simulink model "read_write_sl"  (R2020b)
settings: Solver=VariableStepAuto  StartTime=0.0  StopTime=10.0  RelTol=1e-3
settings Model: Creator=johnc  LastModifiedBy=johnc
settings SFSimCC: SimCustomHeaderCode="#include \"dynamixel_sdk.h\""
settings SFSimCC: SimUserIncludeDirs=|
  | C:\Users\johnc\OneDrive\Documentos\DYNAMIXEL\DynamixelSDK-3.7.31\c\include\dynamixel_sdk\
  | C:\Users\johnc\OneDrive\Documentos\DYNAMIXEL\DynamixelSDK-3.7.31\c\build\win32\output\
  | C:\Users\johnc\OneDrive\Documentos\DYNAMIXEL\DynamixelSDK-3.7.31\c\build\win64\output\
  | C:\Users\johnc\OneDrive\Documentos\DYNAMIXEL\DynamixelSDK-3.7.31\c\src\dynamixel_sdk\
settings SFSimCC: SimUserLibraries=|
  | dxl_x86_c.dll
  | dxl_x64_c.dll
settings SFSimCC: SimUserDefines=|
  | _WIN32
  | _WIN64
  | _cplusplus
  | size_t=unsigned __int64
  | size_t=unsigned in

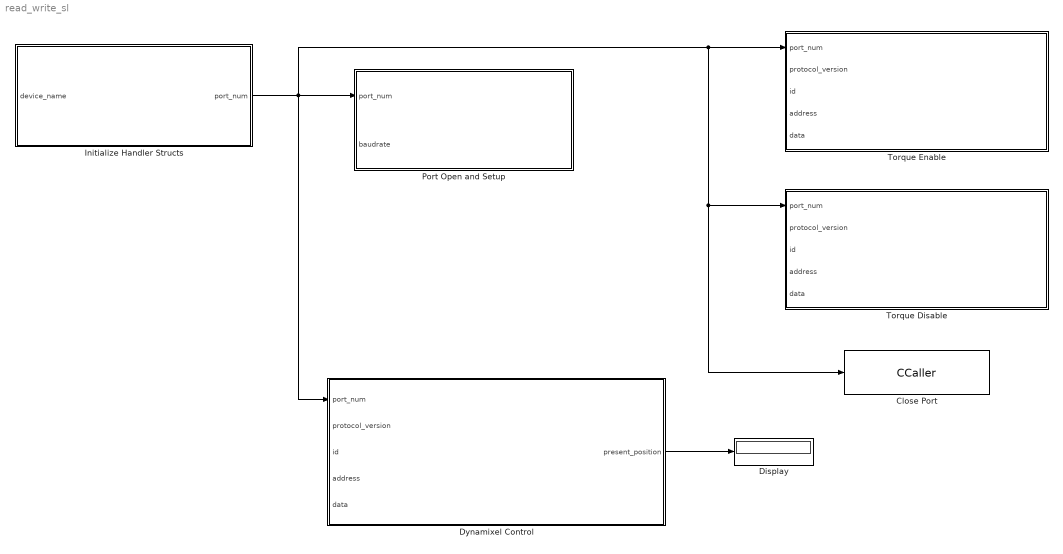
== system read_write_sl ==
  Close Port : CCaller  FunctionName=closePort  PortSpecificationStruct="%)30     .    * (   8    (     @         %    \"     $    !     0         %  0 \"0    $    _    07)G3F%M90  4&]R=$YA;64 4V-O<&4     26YD97@     5'EP90      4VEZ90      27-';&]B86P   X    X    !@    @    $          4    (     0    @    !         !     (    <&]R=%]N=6T.    .     8    (    !          %    \"     $    (     0         0    \"    '!O<G1?;G5M#@   #@    &    \"     0         !0    @    !    !0    $         $     4   !);G!U=     X    X    !@    @    &          4    (     0    $    !          D    (               .    .     8    (    !          %    \"     $    %     0         0    !0   &EN=#,R    #@   #     &    \"     0         !0    @    !     0    $         $  ! #$    .    ,     8    (    \"0(        %    \"     $    !     0         \"  $"
  Display : Display
  Dynamixel Control : Subsystem
  Initialize Handler Structs : Subsystem
  Port Open and Setup : Subsystem
  Torque Disable : Subsystem
  Torque Enable : Subsystem
  wires:
  Initialize Handler Structs/1(port_num) -> Port Open and Setup/1(port_num), Close Port/1, Torque Disable/1(port_num), Torque Enable/1(port_num), Dynamixel Control/1(port_num)
  Dynamixel Control/1(present_position) -> Display/1

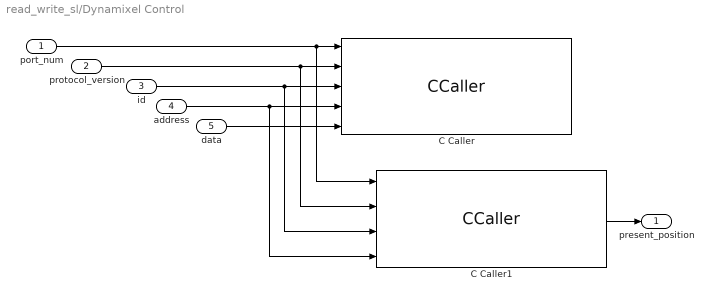
== system read_write_sl/Dynamixel Control ==
  port_num : Inport
  protocol_version : Inport  Port=2
  id : Inport  Port=3
  address : Inport  Port=4
  data : Inport  Port=5
  C Caller : CCaller  FunctionName=write1ByteTxRx  PortSpecificationStruct="%)30     .    V @   8    (     @         %    \"     4    !     0         %  0 \"0    $    _    07)G3F%M90  4&]R=$YA;64 4V-O<&4     26YD97@     5'EP90      4VEZ90      27-';&]B86P   X    X    !@    @    $          4    (     0    @    !         !     (    <&]R=%]N=6T.    .     8    (    !          %    \"     $    (     0         0    \"    '!O<G1?;G5M#@   #@    &    \"     0         !0    @    !  ...(+2668 chars)"
  C Caller1 : CCaller  FunctionName=read2ByteTxRx  PortSpecificationStruct="%)30     .    V @   8    (     @         %    \"     4    !     0         %  0 \"0    $    _    07)G3F%M90  4&]R=$YA;64 4V-O<&4     26YD97@     5'EP90      4VEZ90      27-';&]B86P   X    P    !@    @    $          4    (     0    ,    !         !   P!O=70 #@   #     &    \"     0         !0    @    !     P    $         $  # &]U=  .    .     8    (    !          %    \"     $    &     0         0   ...(+2666 chars)"
  present_position : Outport
  wires:
  port_num/1 -> C Caller1/1, C Caller/1
  address/1 -> C Caller1/4, C Caller/4
  protocol_version/1 -> C Caller1/2, C Caller/2
  id/1 -> C Caller1/3, C Caller/3
  C Caller1/1 -> present_position/1
  data/1 -> C Caller/5

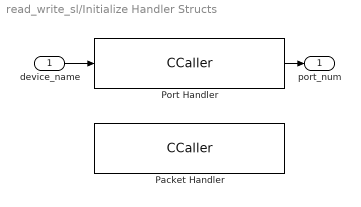
== system read_write_sl/Initialize Handler Structs ==
  device_name : Inport
  Packet Handler : CCaller  FunctionName=packetHandler
  Port Handler : CCaller  FunctionName=portHandler  PortSpecificationStruct="%)30     .    T ,   8    (     @         %    \"     (    !     0         %  0 \"0    $    _    07)G3F%M90  4&]R=$YA;64 4V-O<&4     26YD97@     5'EP90      4VEZ90      27-';&]B86P   X    P    !@    @    $          4    (     0    ,    !         !   P!O=70 #@   #     &    \"     0         !0    @    !     P    $         $  # &]U=  .    .     8    (    !          %    \"     $    &     0         0    !@   $]U='!U=   #@   #@    &    \"     8         !0    @    !     0    $         \"0    @               X    X    !@    @    $          4    (     0    4    !         !     %    :6YT,S(    .    ,     8    (    !          %    \"     $    !     0         0  $ ,0    X    P    !@    @    ) @        4    (     0    $    !          (  0      #@   $     &    \"     0         !0    @    !    \"0    $         $     D   !P;W)T7VYA;64         #@   $     &    \"     0         !0    @    !    \"0    $         $     D   !P;W)T7VYA;64         #@   #@    &    \"     0         !0    @    !    !0    $         $     4   !);G!U=     X    X    !@    @    &          4    (     0    $    !          D    (               .    ,     8    (    !          %    \"     $    $     0         0  0 :6YT. X    P    !@    @    $          4    (     0    (    !         !   @ M,0  #@   #     &    \"     D\"        !0    @    !     0    $          @ !"
  port_num : Outport
  wires:
  device_name/1 -> Port Handler/1
  Port Handler/1 -> port_num/1

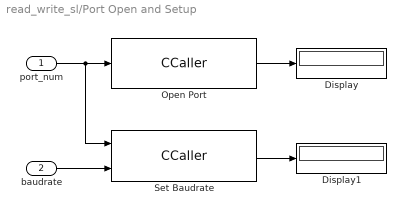
== system read_write_sl/Port Open and Setup ==
  port_num : Inport
  baudrate : Inport  Port=2
  Display : Display
  Display1 : Display
  Open Port : CCaller  FunctionName=openPort  PortSpecificationStruct="%)30     .    R ,   8    (     @         %    \"     (    !     0         %  0 \"0    $    _    07)G3F%M90  4&]R=$YA;64 4V-O<&4     26YD97@     5'EP90      4VEZ90      27-';&]B86P   X    P    !@    @    $          4    (     0    ,    !         !   P!O=70 #@   #     &    \"     0         !0    @    !     P    $         $  # &]U=  .    .     8    (    !          %    \"     $    &     0         0    !@   $]U='!U=   #@   #@    &    \"     8         !0    @    !     0    $         \"0    @               X    X    !@    @    $          4    (     0    4    !         !     %    =6EN=#@    .    ,     8    (    !          %    \"     $    !     0         0  $ ,0    X    P    !@    @    ) @        4    (     0    $    !          (  0      #@   #@    &    \"     0         !0    @    !    \"     $         $     @   !P;W)T7VYU;0X    X    !@    @    $          4    (     0    @    !         !     (    <&]R=%]N=6T.    .     8    (    !          %    \"     $    %     0         0    !0   $EN<'5T    #@   #@    &    \"     8         !0    @    !     0    $         \"0    @               X    X    !@    @    $          4    (     0    4    !         !     %    :6YT,S(    .    ,     8    (    !          %    \"     $    !     0         0  $ ,0    X    P    !@    @    ) @        4    (     0    $    !          (  0"
  Set Baudrate : CCaller  FunctionName=setBaudRate  PortSpecificationStruct="%)30     .    > 4   8    (     @         %    \"     ,    !     0         %  0 \"0    $    _    07)G3F%M90  4&]R=$YA;64 4V-O<&4     26YD97@     5'EP90      4VEZ90      27-';&]B86P   X    P    !@    @    $          4    (     0    ,    !         !   P!O=70 #@   #     &    \"     0         !0    @    !     P    $         $  # &]U=  .    .     8    (    !          %    \"     $    &     0         0    !@   $]U='!U=   #@   #@    &    \"     8         !0    @    !     0    $         \"0    @               X    X    !@    @    $          4    (     0    4    !         !     %    =6EN=#@    .    ,     8    (    !          %    \"     $    !     0         0  $ ,0    X    P    !@    @    ) @        4    (     0    $    !          (  0      #@   #@    &    \"     0         !0    @    !    \"     $         $     @   !P;W)T7VYU;0X    X    !@    @    $          4    (     0    @    !         !     (    <&]R=%]N=6T.    .     8    (    !          %    \"     $    %     0         0    !0   $EN<'5T    #@   #@    &    \"     8         !0    @    !     0    $         \"0    @               X    X    !@    @    $          4    (     0    4    !         !     %    :6YT,S(    .    ,     8    (    !          %    \"     $    !     0         0  $ ,0    X    P    !@    @    ) @        4    (     0    $    !          (  0      #@   #@    &    \"     0         !0    @    !    \"     $         $     @   !B875D<F%T90X    X    !@    @    $          4    (     0    @    !         !     (    8F%U9')A=&4.    .     8    (    !          %    \"     $    %     0         0    !0   $EN<'5T    #@   #@    &    \"     8         !0    @    !     0    $         \"0    @           #P/PX    X    !@    @    $          4    (     0    4    !         !     %    :6YT,S(    .    ,     8    (    !          %    \"     $    !     0         0  $ ,0    X    P    !@    @    ) @        4    (     0    $    !          (  0"
  wires:
  baudrate/1 -> Set Baudrate/2
  Open Port/1 -> Display/1
  Set Baudrate/1 -> Display1/1
  port_num/1 -> Set Baudrate/1, Open Port/1

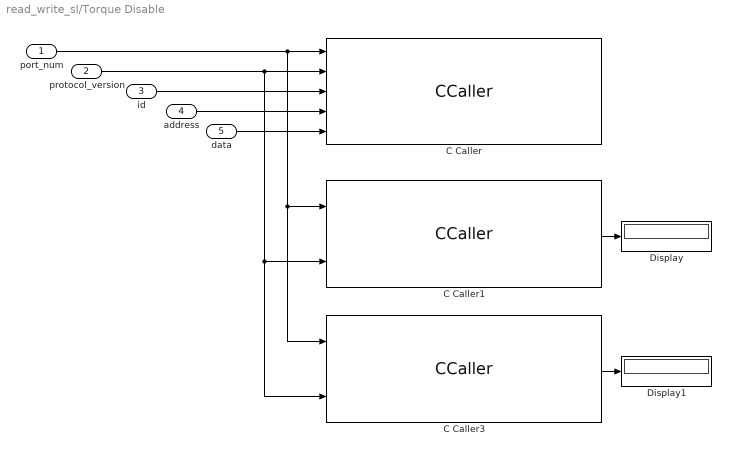
== system read_write_sl/Torque Disable ==
  port_num : Inport
  protocol_version : Inport  Port=2
  id : Inport  Port=3
  address : Inport  Port=4
  data : Inport  Port=5
  C Caller : CCaller  FunctionName=write1ByteTxRx  PortSpecificationStruct="%)30     .    V @   8    (     @         %    \"     4    !     0         %  0 \"0    $    _    07)G3F%M90  4&]R=$YA;64 4V-O<&4     26YD97@     5'EP90      4VEZ90      27-';&]B86P   X    X    !@    @    $          4    (     0    @    !         !     (    <&]R=%]N=6T.    .     8    (    !          %    \"     $    (     0         0    \"    '!O<G1?;G5M#@   #@    &    \"     0         !0    @    !  ...(+2668 chars)"
  C Caller1 : CCaller  FunctionName=getLastTxRxResult  PortSpecificationStruct="%)30     .    B 4   8    (     @         %    \"     ,    !     0         %  0 \"0    $    _    07)G3F%M90  4&]R=$YA;64 4V-O<&4     26YD97@     5'EP90      4VEZ90      27-';&]B86P   X    P    !@    @    $          4    (     0    ,    !         !   P!O=70 #@   #     &    \"     0         !0    @    !     P    $         $  # &]U=  .    .     8    (    !          %    \"     $    &     0         0    !@   $]U='!U=   #@   #@    &    \"     8         !0    @    !     0    $         \"0    @               X    X    !@    @    $          4    (     0    4    !         !     %    :6YT,S(    .    ,     8    (    !          %    \"     $    !     0         0  $ ,0    X    P    !@    @    ) @        4    (     0    $    !          (  0      #@   #@    &    \"     0         !0    @    !    \"     $         $     @   !P;W)T7VYU;0X    X    !@    @    $          4    (     0    @    !         !     (    <&]R=%]N=6T.    .     8    (    !          %    \"     $    %     0         0    !0   $EN<'5T    #@   #@    &    \"     8         !0    @    !     0    $         \"0    @               X    X    !@    @    $          4    (     0    4    !         !     %    :6YT,S(    .    ,     8    (    !          %    \"     $    !     0         0  $ ,0    X    P    !@    @    ) @        4    (     0    $    !          (  0      #@   $     &    \"     0         !0    @    !    $     $         $    !    !P<F]T;V-O;%]V97)S:6]N#@   $     &    \"     0         !0    @    !    $     $         $    !    !P<F]T;V-O;%]V97)S:6]N#@   #@    &    \"     0         !0    @    !    !0    $         $     4   !);G!U=     X    X    !@    @    &          4    (     0    $    !          D    (            \\#\\.    .     8    (    !          %    \"     $    %     0         0    !0   &EN=#,R    #@   #     &    \"     0         !0    @    !     0    $         $  ! #$    .    ,     8    (    \"0(        %    \"     $    !     0         \"  $"
  C Caller3 : CCaller  FunctionName=getLastRxPacketError  PortSpecificationStruct="%)30     .    B 4   8    (     @         %    \"     ,    !     0         %  0 \"0    $    _    07)G3F%M90  4&]R=$YA;64 4V-O<&4     26YD97@     5'EP90      4VEZ90      27-';&]B86P   X    P    !@    @    $          4    (     0    ,    !         !   P!O=70 #@   #     &    \"     0         !0    @    !     P    $         $  # &]U=  .    .     8    (    !          %    \"     $    &     0         0    !@   $]U='!U=   #@   #@    &    \"     8         !0    @    !     0    $         \"0    @               X    X    !@    @    $          4    (     0    4    !         !     %    =6EN=#@    .    ,     8    (    !          %    \"     $    !     0         0  $ ,0    X    P    !@    @    ) @        4    (     0    $    !          (  0      #@   #@    &    \"     0         !0    @    !    \"     $         $     @   !P;W)T7VYU;0X    X    !@    @    $          4    (     0    @    !         !     (    <&]R=%]N=6T.    .     8    (    !          %    \"     $    %     0         0    !0   $EN<'5T    #@   #@    &    \"     8         !0    @    !     0    $         \"0    @               X    X    !@    @    $          4    (     0    4    !         !     %    :6YT,S(    .    ,     8    (    !          %    \"     $    !     0         0  $ ,0    X    P    !@    @    ) @        4    (     0    $    !          (  0      #@   $     &    \"     0         !0    @    !    $     $         $    !    !P<F]T;V-O;%]V97)S:6]N#@   $     &    \"     0         !0    @    !    $     $         $    !    !P<F]T;V-O;%]V97)S:6]N#@   #@    &    \"     0         !0    @    !    !0    $         $     4   !);G!U=     X    X    !@    @    &          4    (     0    $    !          D    (            \\#\\.    .     8    (    !          %    \"     $    %     0         0    !0   &EN=#,R    #@   #     &    \"     0         !0    @    !     0    $         $  ! #$    .    ,     8    (    \"0(        %    \"     $    !     0         \"  $"
  Display : Display
  Display1 : Display
  wires:
  data/1 -> C Caller/5
  id/1 -> C Caller/3
  C Caller3/1 -> Display1/1
  address/1 -> C Caller/4
  protocol_version/1 -> C Caller/2, C Caller1/2, C Caller3/2
  C Caller1/1 -> Display/1
  port_num/1 -> C Caller/1, C Caller1/1, C Caller3/1

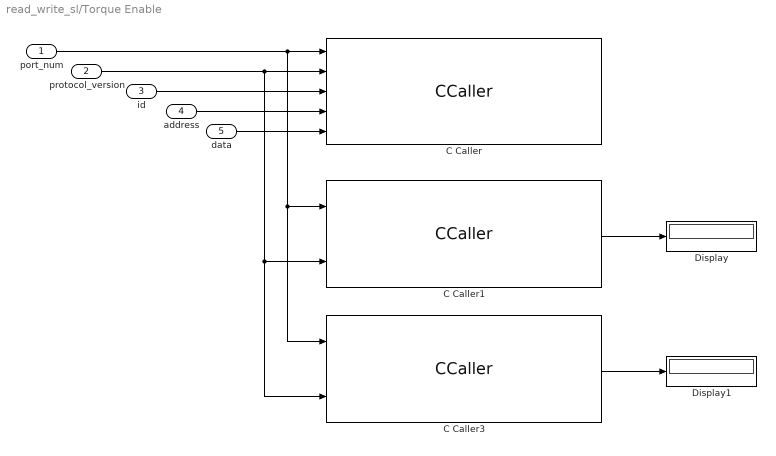
== system read_write_sl/Torque Enable ==
  port_num : Inport
  protocol_version : Inport  Port=2
  id : Inport  Port=3
  address : Inport  Port=4
  data : Inport  Port=5
  C Caller : CCaller  FunctionName=write1ByteTxRx  PortSpecificationStruct="%)30     .    V @   8    (     @         %    \"     4    !     0         %  0 \"0    $    _    07)G3F%M90  4&]R=$YA;64 4V-O<&4     26YD97@     5'EP90      4VEZ90      27-';&]B86P   X    X    !@    @    $          4    (     0    @    !         !     (    <&]R=%]N=6T.    .     8    (    !          %    \"     $    (     0         0    \"    '!O<G1?;G5M#@   #@    &    \"     0         !0    @    !  ...(+2668 chars)"
  C Caller1 : CCaller  FunctionName=getLastTxRxResult  PortSpecificationStruct="%)30     .    B 4   8    (     @         %    \"     ,    !     0         %  0 \"0    $    _    07)G3F%M90  4&]R=$YA;64 4V-O<&4     26YD97@     5'EP90      4VEZ90      27-';&]B86P   X    P    !@    @    $          4    (     0    ,    !         !   P!O=70 #@   #     &    \"     0         !0    @    !     P    $         $  # &]U=  .    .     8    (    !          %    \"     $    &     0         0    !@   $]U='!U=   #@   #@    &    \"     8         !0    @    !     0    $         \"0    @               X    X    !@    @    $          4    (     0    4    !         !     %    :6YT,S(    .    ,     8    (    !          %    \"     $    !     0         0  $ ,0    X    P    !@    @    ) @        4    (     0    $    !          (  0      #@   #@    &    \"     0         !0    @    !    \"     $         $     @   !P;W)T7VYU;0X    X    !@    @    $          4    (     0    @    !         !     (    <&]R=%]N=6T.    .     8    (    !          %    \"     $    %     0         0    !0   $EN<'5T    #@   #@    &    \"     8         !0    @    !     0    $         \"0    @               X    X    !@    @    $          4    (     0    4    !         !     %    :6YT,S(    .    ,     8    (    !          %    \"     $    !     0         0  $ ,0    X    P    !@    @    ) @        4    (     0    $    !          (  0      #@   $     &    \"     0         !0    @    !    $     $         $    !    !P<F]T;V-O;%]V97)S:6]N#@   $     &    \"     0         !0    @    !    $     $         $    !    !P<F]T;V-O;%]V97)S:6]N#@   #@    &    \"     0         !0    @    !    !0    $         $     4   !);G!U=     X    X    !@    @    &          4    (     0    $    !          D    (            \\#\\.    .     8    (    !          %    \"     $    %     0         0    !0   &EN=#,R    #@   #     &    \"     0         !0    @    !     0    $         $  ! #$    .    ,     8    (    \"0(        %    \"     $    !     0         \"  $"
  C Caller3 : CCaller  FunctionName=getLastRxPacketError  PortSpecificationStruct="%)30     .    B 4   8    (     @         %    \"     ,    !     0         %  0 \"0    $    _    07)G3F%M90  4&]R=$YA;64 4V-O<&4     26YD97@     5'EP90      4VEZ90      27-';&]B86P   X    P    !@    @    $          4    (     0    ,    !         !   P!O=70 #@   #     &    \"     0         !0    @    !     P    $         $  # &]U=  .    .     8    (    !          %    \"     $    &     0         0    !@   $]U='!U=   #@   #@    &    \"     8         !0    @    !     0    $         \"0    @               X    X    !@    @    $          4    (     0    4    !         !     %    =6EN=#@    .    ,     8    (    !          %    \"     $    !     0         0  $ ,0    X    P    !@    @    ) @        4    (     0    $    !          (  0      #@   #@    &    \"     0         !0    @    !    \"     $         $     @   !P;W)T7VYU;0X    X    !@    @    $          4    (     0    @    !         !     (    <&]R=%]N=6T.    .     8    (    !          %    \"     $    %     0         0    !0   $EN<'5T    #@   #@    &    \"     8         !0    @    !     0    $         \"0    @               X    X    !@    @    $          4    (     0    4    !         !     %    :6YT,S(    .    ,     8    (    !          %    \"     $    !     0         0  $ ,0    X    P    !@    @    ) @        4    (     0    $    !          (  0      #@   $     &    \"     0         !0    @    !    $     $         $    !    !P<F]T;V-O;%]V97)S:6]N#@   $     &    \"     0         !0    @    !    $     $         $    !    !P<F]T;V-O;%]V97)S:6]N#@   #@    &    \"     0         !0    @    !    !0    $         $     4   !);G!U=     X    X    !@    @    &          4    (     0    $    !          D    (            \\#\\.    .     8    (    !          %    \"     $    %     0         0    !0   &EN=#,R    #@   #     &    \"     0         !0    @    !     0    $         $  ! #$    .    ,     8    (    \"0(        %    \"     $    !     0         \"  $"
  Display : Display
  Display1 : Display
  wires:
  port_num/1 -> C Caller3/1, C Caller1/1, C Caller/1
  C Caller1/1 -> Display/1
  protocol_version/1 -> C Caller3/2, C Caller1/2, C Caller/2
  address/1 -> C Caller/4
  C Caller3/1 -> Display1/1
  id/1 -> C Caller/3
  data/1 -> C Caller/5
